simulink model "pacemaker_ass2_test_Reaction_Time"  (R2017b)
settings: Solver=FixedStepAuto  StartTime=0.0  StopTime=inf  FixedStep=0.001  RelTol=1e-3  EnableMultiTasking=on
libraries: frdmk64flib x4
settings Model: ExtModeTrigDuration=5  Creator=montema2  LastModifiedBy=montema2
settings SolverCC: AutoInsertRateTranBlk=on
settings DataIOCC: LimitDataPoints=on
settings OptimizationCC: PassReuseOutputArgsAs=Individual arguments  MaxStackSize=64
settings DebuggingCC: ParameterTunabilityLossMsg=error  AllowSymbolicDim=off  SFUnexpectedBacktrackingDiag=warning  SFNoUnconditionalDefaultTransitionDiag=warning  SFExecutionAtInitializationDiag=none
settings HardwareCC: ProdBitPerPointer=32  ProdBitPerSizeT=32  ProdBitPerPtrDiffT=32  ProdLargestAtomicInteger=Long  ProdLargestAtomicFloat=Double  ProdWordSize=32  ProdHWDeviceType=ARM Compatible->ARM Cortex
settings SFSimCC: MATLABDynamicMemAlloc=off
settings RTWCC: SystemTargetFile=ert.tlc  HardwareBoard=NXP FRDM-K64F  TemplateMakefile=ert_default_tmf  GenerateReport=on  Toolchain=GNU Tools for ARM Embedded Processors  IncludeHyperlinkInReport=on  LaunchReport=on  GenerateTraceInfo=on  GenerateTraceReport=on  GenerateTraceReportSl=on  GenerateTraceReportSf=on  GenerateTraceReportEml=on
settings CodeAppCC: ForceParamTrailComments=on  IgnoreCustomStorageClasses=off  OperatorAnnotations=on  SimulinkDataObjDesc=on  SFDataObjDesc=on  InsertBlockDesc=on
settings ConfigComp: CovMetricSettings=dw  CovHtmlReporting=on  CovSaveCumulativeToWorkspaceVar=on  CovSaveSingleToWorkspaceVar=on  CovShowResultsExplorer=off  CovExternalEMLEnable=off  CovSFcnEnable=off

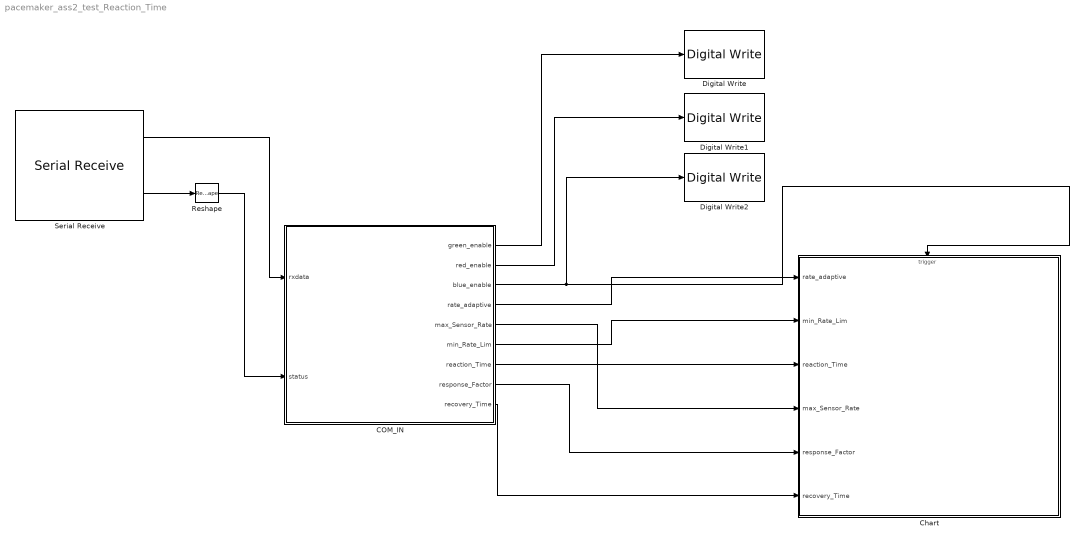
== system pacemaker_ass2_test_Reaction_Time ==
  COM_IN : Stateflow chart  TreatAsAtomicUnit=on
  Chart : Stateflow chart  TreatAsAtomicUnit=on
  Digital Write : frdmk64flib/Digital Write  Whichpin=GREEN_LED
      settings: SourceProductName=Simulink Coder Support Package for NXP FRDM-K64F Board
  Digital Write1 : frdmk64flib/Digital Write  Whichpin=RED_LED
      settings: SourceProductName=Simulink Coder Support Package for NXP FRDM-K64F Board
  Digital Write2 : frdmk64flib/Digital Write  Whichpin=BLUE_LED
      settings: SourceProductName=Simulink Coder Support Package for NXP FRDM-K64F Board
  Reshape : Reshape  OutputDimensionality=Customize  OutputDimensions=[1]
  Serial Receive : frdmk64flib/Serial Receive  SCIModule=0  Baudrate=uint32(9600)  Parity=None  StopBits=1  HardwareFlowControl=None  ByteOrder=LittleEndian  DataType=uint8  DataLength=4  BlockingMode=off  OutputStatus=on  SampleTime=-1
      settings: SourceProductName=Simulink Coder Support Package for NXP FRDM-K64F Board
  wires:
  Serial Receive/2 -> Reshape/1
  COM_IN/1(green_enable) -> Digital Write/1
  Serial Receive/1 -> COM_IN/1(rxdata)
  COM_IN/2(red_enable) -> Digital Write1/1
  Reshape/1 -> COM_IN/2(status)
  COM_IN/4(rate_adaptive) -> Chart/1(rate_adaptive)
  COM_IN/5(max_Sensor_Rate) -> Chart/4(max_Sensor_Rate)
  COM_IN/6(min_Rate_Lim) -> Chart/2(min_Rate_Lim)
  COM_IN/7(reaction_Time) -> Chart/3(reaction_Time)
  COM_IN/8(response_Factor) -> Chart/5(response_Factor)
  COM_IN/3(blue_enable) -> Chart/Trigger, Digital Write2/1
  COM_IN/9(recovery_Time) -> Chart/6(recovery_Time)

== stateflow chart pacemaker_ass2_test_Reaction_Time/Chart ==
  state Spike_Counter_AND_Constant
    entry: rate=min_Rate_Lim;
  state Rate_Increasing
    entry: rate_of_increase=(max_Sensor_Rate/min_Rate_Lim)*response_Factor;
  state Rate_Decreasing_AND_Counting
    entry: rate_of_decrease=((min_Rate_Lim)-(max_Sensor_Rate))/(60*recovery_Time);
  state Increase_rate
    entry: rate = rate + rate_of_increase;
  state Rate_Constant
  (default) -> Spike_Counter_AND_Constant : [rate_adaptive==1]
  Spike_Counter_AND_Constant -> Spike_Counter_AND_Constant [order 1] : [after(reaction_Time,sec)]
  Rate_Decreasing_AND_Counting -> Spike_Counter_AND_Constant [order 1] : [rate<min_Rate_Lim]
  Spike_Counter_AND_Constant -> Rate_Increasing [order 2] : [after(3,spike)]
  Rate_Decreasing_AND_Counting -> Rate_Decreasing_AND_Counting [order 2] : [after(reaction_Time,sec) ]
  Rate_Increasing -> Rate_Increasing [order 3] : [(rate<max_Sensor_Rate) && after(1,spike)]
  Rate_Increasing -> Rate_Decreasing_AND_Counting [order 2] : [after(reaction_Time,sec)]
  Rate_Increasing -> Increase_rate [order 4] : [after(1,sec)]
  Rate_Decreasing_AND_Counting -> Rate_Increasing [order 3] : [after(3,spike)]
  Rate_Constant -> Rate_Decreasing_AND_Counting [order 1] : [after(reaction_Time,sec)]
  Increase_rate -> Rate_Increasing
  Rate_Increasing -> Rate_Constant [order 1] : [(rate>=max_Sensor_Rate) && after (1,spike)]
  Rate_Constant -> Rate_Constant [order 2] : [after(1,spike)]
  data: rate_adaptive input; min_Rate_Lim input; reaction_Time input; max_Sensor_Rate input; response_Factor input; recovery_Time input; rate_of_decrease local; rate_of_increase local; rate local
  events: spike input RISING_EDGE_EVENT

== stateflow chart pacemaker_ass2_test_Reaction_Time/COM_IN ==
  settings: executeAtInitialization=1
  state INITIAL
    entry:
    red_enable = 0;
    green_enable = 0;
    blue_enable = 0;
    rate_adaptive=1;
    min_Rate_Lim=60;
    reaction_Time=2;
    max_Sensor_Rate=120;
    response_Factor=1;
    recovery_Time=1;
  state STANDBY
    entry:
    green_enable = 0;
    red_enable = 0;
    blue_enable = 1;
  state state
    entry:
    green_enable = 0;
    red_enable = 1;
    blue_enable = 0;
  state state2
    entry:
    red_enable = 0;
    green_enable = 1;
    blue_enable = 0;
  state -> STANDBY : [after(1000,msec)]
  (default) -> INITIAL
  INITIAL -> STANDBY
  STANDBY -> (junction 11) : [status == 0]
  (junction 11) -> state [order 1] : [typecast(rxdata(1:2),'int16') == 22 && typecast(rxdata(3:4),'int16') == 4]
  (junction 11) -> state2 [order 2]
  (junction 11) -> state2 [commented out] : [typecast(rxdata(3:4),'int16') == 14]
  state2 -> STANDBY : [after(1000,msec)]
  data: rxdata input uint8; status input uint8; green_enable output; red_enable output; blue_enable output; rate_adaptive output; max_Sensor_Rate output; min_Rate_Lim output; reaction_Time output; response_Factor output; recovery_Time output
